simulink model "PTC_MBDS_StringLen_Sample"  (R2013a)
settings: Solver=FixedStepDiscrete  StartTime=0.0  StopTime=100  FixedStep=0.02  RelTol=1e-3
undefined symbols (not defined in the file): ptc_matlab_lib
libraries: simulink_extras x3, PTC_MBDS_LIB x3
settings Model: Creator=uidl7367  LastModifiedBy=sundeep.tuteja
settings DataIOCC: SignalLoggingSaveFormat=ModelDataLogs
settings OptimizationCC: ExpressionDepthLimit=2147483647  InitFltsAndDblsToZero=on
settings DebuggingCC: SaveWithParameterizedLinksMsg=none  SignalResolutionControl=TryResolveAllWithWarning  SolverPrmCheckMsg=none  InheritedTsInSrcMsg=none  MultiTaskDSMMsg=warning  MultiTaskCondExecSysMsg=none  FcnCallInpInsideContextMsg=UseLocalSettings  StrictBusMsg=Warning
settings RTWCC: IncludeERTFirstTime=on
settings GRTTargetCC: TargetFcnLib=ansi_tfl_tmw.mat  CombineOutputUpdateFcns=off  GRTInterface=on

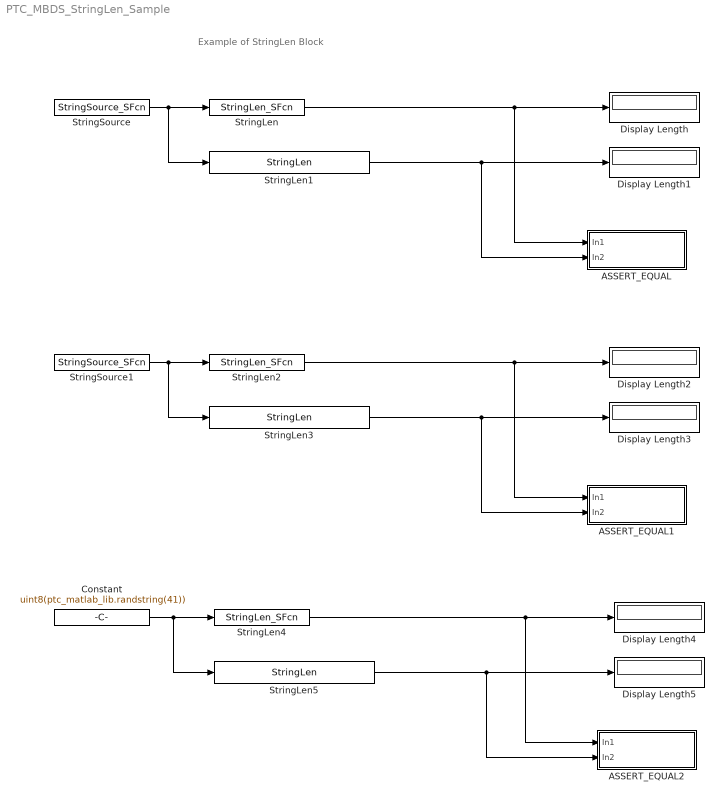
== system PTC_MBDS_StringLen_Sample ==
  note: Example of StringLen Block
  ASSERT_EQUAL : Subsystem
  ASSERT_EQUAL1 : Subsystem
  ASSERT_EQUAL2 : Subsystem
  Constant : Constant  Value=uint8(ptc_matlab_lib.randstring(41))
  Display Length{,1..5} (6 alike) : Display
  StringLen : S-Function  InitFcn=|  FunctionName=StringLen_SFcn  Parameters=uint16(MaxStringLength)  EnableBusSupport=off  mask(StringLen){MBDS_LibraryBlock=on, MBDS_BlockVersion=05.40}
      | if(exist('MBDS_BlockCallback', 'file'))
      |    MBDS_BlockCallback('Update', gcb);
      | end
      mask prompts: MBDS_LibraryBlock "MBDS Library Block"; MBDS_BlockVersion "Block version:"
      mask help: Determines the length of a string signal.
      mask init:
      | MBDS_BlockCallback('Copy', gcb);
      | MaxStringLength = 1 + GetStringLen();
      mask Help: eval(['open([workdir(''Library_Dir:''),''\Blockset\Help\'',get_param(gcb,''MaskType''),''.html''])'])
      mask Display:
      | disp('Len')
      | port_label('input', 1, 'In')
      | port_label('output', 1, 'Out')
  StringLen1 : PTC_MBDS_LIB/MBDS Standard Library/Extended Operations/String Operations/StringLen  PTC_MBDS_BlockVersion=5.32  PTC_BlockType=PTC_MBDS_StringLen  MaxStringLength=PTC_MBDS_MaxStringLength_Fcn
  StringLen2 : S-Function  InitFcn=|  FunctionName=StringLen_SFcn  Parameters=uint16(MaxStringLength)  EnableBusSupport=off  mask(StringLen){MBDS_LibraryBlock=on, MBDS_BlockVersion=05.40}
      | if(exist('MBDS_BlockCallback', 'file'))
      |    MBDS_BlockCallback('Update', gcb);
      | end
      mask prompts: MBDS_LibraryBlock "MBDS Library Block"; MBDS_BlockVersion "Block version:"
      mask help: Determines the length of a string signal.
      mask init:
      | MBDS_BlockCallback('Copy', gcb);
      | MaxStringLength = 1 + GetStringLen();
      mask Help: eval(['open([workdir(''Library_Dir:''),''\Blockset\Help\'',get_param(gcb,''MaskType''),''.html''])'])
      mask Display:
      | disp('Len')
      | port_label('input', 1, 'In')
      | port_label('output', 1, 'Out')
  StringLen3 : PTC_MBDS_LIB/MBDS Standard Library/Extended Operations/String Operations/StringLen  PTC_MBDS_BlockVersion=5.32  PTC_BlockType=PTC_MBDS_StringLen  MaxStringLength=PTC_MBDS_MaxStringLength_Fcn
  StringLen4 : S-Function  InitFcn=|  FunctionName=StringLen_SFcn  Parameters=uint16(MaxStringLength)  EnableBusSupport=off  mask(StringLen){MBDS_LibraryBlock=on, MBDS_BlockVersion=05.40}
      | if(exist('MBDS_BlockCallback', 'file'))
      |    MBDS_BlockCallback('Update', gcb);
      | end
      mask prompts: MBDS_LibraryBlock "MBDS Library Block"; MBDS_BlockVersion "Block version:"
      mask help: Determines the length of a string signal.
      mask init:
      | MBDS_BlockCallback('Copy', gcb);
      | MaxStringLength = 1 + GetStringLen();
      mask Help: eval(['open([workdir(''Library_Dir:''),''\Blockset\Help\'',get_param(gcb,''MaskType''),''.html''])'])
      mask Display:
      | disp('Len')
      | port_label('input', 1, 'In')
      | port_label('output', 1, 'Out')
  StringLen5 : PTC_MBDS_LIB/MBDS Standard Library/Extended Operations/String Operations/StringLen  PTC_MBDS_BlockVersion=5.32  PTC_BlockType=PTC_MBDS_StringLen  MaxStringLength=PTC_MBDS_MaxStringLength_Fcn
  StringSource : S-Function  InitFcn=|  FunctionName=StringSource_SFcn  Parameters=uint8(String), uint16(MaxStringLength)  EnableBusSupport=off  mask(StringSource){MBDS_LibraryBlock=on, InputValue=aaaaaaaaaaaaaaaaaaaaaaaaaaaaaaaaaaaaaaaa, MBDS_BlockVersion=05.20}
      | if(exist('MBDS_BlockCallback', 'file'))
      |    MBDS_BlockCallback('Update', gcb);
      | end
      mask prompts: MBDS_LibraryBlock "MBDS Library Block"; InputValue "Constant value:"; MBDS_BlockVersion "Block version:"
      mask help: This block outputs an uint8 array based on the ASCII codes of the string specified by the user.
      mask init:
      | MBDS_BlockCallback('Copy', gcb);
      | MaxStringLength = 1 + GetStringLen();
      | DispString = 'Error';
      | String = InputValue;
      | % Skip if string specifies a numeric expression or starts with '
      | if(isempty(str2num(String)) && String(1) ~= '''')
      |    try
      |       % Try to evaluate project constant 
      |       String = evalin('base', String);
      |    end   
      | end
      | if ~ischar(String) || size(String, 1) > 1
      | 	error('String must be a [1xn] array of type ''char'' with at least one character')
      | else
      |    % Limit to max. string length
      |    String = String(1:min(MaxStringLength, length(String)));
      | 	DispString = InputValue;
      | end
      mask Help: eval(['open([workdir(''Library_Dir:''),''\Blockset\Help\'',get_param(gcb,''MaskType''),''.html''])'])
      mask Display: text(0.05,0.5,DispString,'horizontalAlignment','left')
  StringSource1 : S-Function  InitFcn=|  FunctionName=StringSource_SFcn  Parameters=uint8(String), uint16(MaxStringLength)  EnableBusSupport=off  mask(StringSource){MBDS_LibraryBlock=on, InputValue=4gjh, MBDS_BlockVersion=05.20}
      | if(exist('MBDS_BlockCallback', 'file'))
      |    MBDS_BlockCallback('Update', gcb);
      | end
      mask prompts: MBDS_LibraryBlock "MBDS Library Block"; InputValue "Constant value:"; MBDS_BlockVersion "Block version:"
      mask help: This block outputs an uint8 array based on the ASCII codes of the string specified by the user.
      mask init: same as PTC_MBDS_StringLen_Sample/StringSource
      mask Help: eval(['open([workdir(''Library_Dir:''),''\Blockset\Help\'',get_param(gcb,''MaskType''),''.html''])'])
      mask Display: text(0.05,0.5,DispString,'horizontalAlignment','left')
  wires:
  StringLen/1 -> ASSERT_EQUAL/1(In1), Display Length/1
  StringSource/1 -> StringLen/1, StringLen1/1
  StringLen1/1 -> ASSERT_EQUAL/2(In2), Display Length1/1
  StringLen2/1 -> Display Length2/1, ASSERT_EQUAL1/1(In1)
  StringSource1/1 -> StringLen2/1, StringLen3/1
  StringLen3/1 -> Display Length3/1, ASSERT_EQUAL1/2(In2)
  StringLen4/1 -> ASSERT_EQUAL2/1(In1), Display Length4/1
  Constant/1 -> StringLen4/1, StringLen5/1
  StringLen5/1 -> ASSERT_EQUAL2/2(In2), Display Length5/1

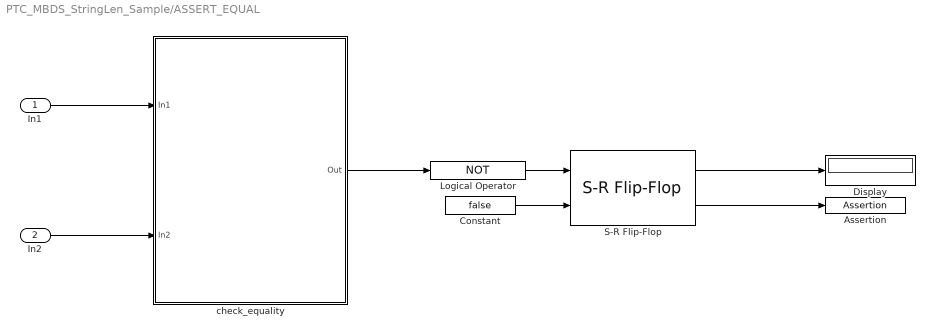
== system PTC_MBDS_StringLen_Sample/ASSERT_EQUAL ==
  In1 : Inport
  In2 : Inport  Port=2
  Assertion : Assertion
  Constant : Constant  Value=false
  Display : Display
  Logical Operator : Logic  Operator=NOT  AllPortsSameDT=off  OutDataTypeStr=boolean
  S-R Flip-Flop : simulink_extras/Flip Flops/S-R Flip-Flop  initial_condition=0
  check_equality : MATLAB Function  TreatAsAtomicUnit=on
  wires:
  S-R Flip-Flop/1 -> Display/1
  check_equality/1(Out) -> Logical Operator/1
  Constant/1 -> S-R Flip-Flop/2
  S-R Flip-Flop/2 -> Assertion/1
  In2/1 -> check_equality/2(In2)
  In1/1 -> check_equality/1(In1)
  Logical Operator/1 -> S-R Flip-Flop/1

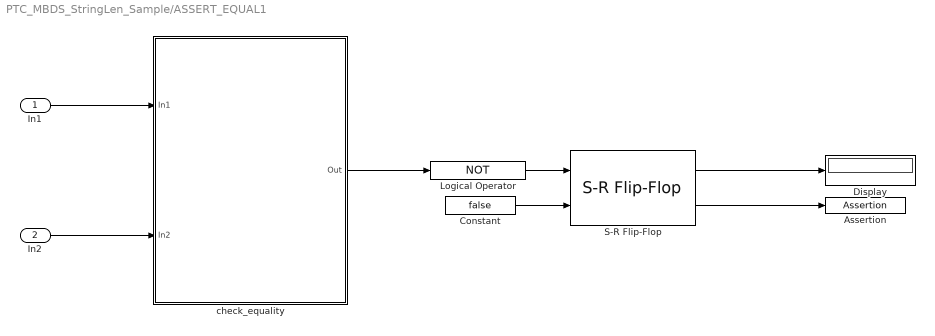
== system PTC_MBDS_StringLen_Sample/ASSERT_EQUAL1 ==
  In1 : Inport
  In2 : Inport  Port=2
  Assertion : Assertion
  Constant : Constant  Value=false
  Display : Display
  Logical Operator : Logic  Operator=NOT  AllPortsSameDT=off  OutDataTypeStr=boolean
  S-R Flip-Flop : simulink_extras/Flip Flops/S-R Flip-Flop  initial_condition=0
  check_equality : MATLAB Function  TreatAsAtomicUnit=on
  wires:
  Logical Operator/1 -> S-R Flip-Flop/1
  In1/1 -> check_equality/1(In1)
  In2/1 -> check_equality/2(In2)
  S-R Flip-Flop/2 -> Assertion/1
  Constant/1 -> S-R Flip-Flop/2
  check_equality/1(Out) -> Logical Operator/1
  S-R Flip-Flop/1 -> Display/1

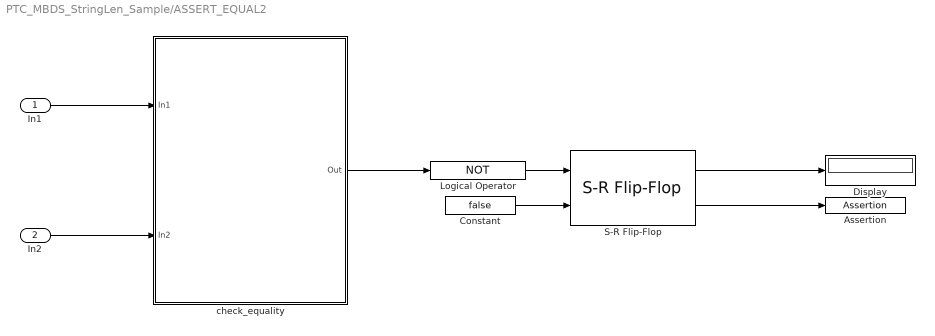
== system PTC_MBDS_StringLen_Sample/ASSERT_EQUAL2 ==
  In1 : Inport
  In2 : Inport  Port=2
  Assertion : Assertion
  Constant : Constant  Value=false
  Display : Display
  Logical Operator : Logic  Operator=NOT  AllPortsSameDT=off  OutDataTypeStr=boolean
  S-R Flip-Flop : simulink_extras/Flip Flops/S-R Flip-Flop  initial_condition=0
  check_equality : MATLAB Function  TreatAsAtomicUnit=on
  wires:
  Logical Operator/1 -> S-R Flip-Flop/1
  In1/1 -> check_equality/1(In1)
  In2/1 -> check_equality/2(In2)
  S-R Flip-Flop/2 -> Assertion/1
  Constant/1 -> S-R Flip-Flop/2
  check_equality/1(Out) -> Logical Operator/1
  S-R Flip-Flop/1 -> Display/1

== matlab function PTC_MBDS_StringLen_Sample/ASSERT_EQUAL1/check_equality ==
  data: In1 input; Out output; In2 input
function Out = check_equality(In1, In2)
%#codegen

Out = isequaln(In1, In2);

end

== matlab function PTC_MBDS_StringLen_Sample/ASSERT_EQUAL/check_equality ==
  data: In1 input; Out output; In2 input
function Out = check_equality(In1, In2)
%#codegen

Out = isequaln(In1, In2);

end

== matlab function PTC_MBDS_StringLen_Sample/ASSERT_EQUAL2/check_equality ==
  data: In1 input; Out output; In2 input
function Out = check_equality(In1, In2)
%#codegen

Out = isequaln(In1, In2);

end
